simulink model "gm_soc_dvbs2_fpga"  (R2025b)
settings: Solver=VariableStepAuto  StartTime=0.0  StopTime=10.0  RelTol=1e-3
InitFcn:
  | soc_dvbs2_init;
undefined symbols (not defined in the file or in its folder): Add, coefficientsLog, coefficientsSqrt1, coefficientsSqrt2, dataBits, Deinterleaver, designMultirateFIR, noisePow, Shift, Short, soc_dvbs2_designFIRFilter, soc_dvbs2_txPacketBits, syncWord, txDataOut, txFiltCoeff, XData
libraries: simulink x304, hdlsllib x265, dspsigops x15, dsphdlfiltering2 x8, hdlmdlgenlib x6, dsphdlsigops2 x5, commseqgen3 x5, dsphdlmathfun2 x3, hwlogicconnlib x2, whdledac x2, commhdlcrc x2, whdlutilities x1
(part 35 of 36)

== system gm_soc_dvbs2_fpga/DVBS2/DVBS2 TxRx/DVB-S2 HDL Receiver/Synchronizer and PL Header Decoder/Time Frequency and Coarse Phase Synchronizer/Fine Frequency Synchronizer/Modified L and R Algorithm/L and R Algorithm 18 point/Compute R(m) for 7 to 12/Compute R(m)_1 ==
  z : Inport  OutDataTypeStr=fixdt(1, 16, 11)  PortDimensions=1  SampleTime=2.5e-07
      settings: SignalType=complex
  zvalid : Inport  Port=2  OutDataTypeStr=boolean  PortDimensions=1  SampleTime=2.5e-07
  Add3 : Sum  OutDataTypeStr=fixdt(1, 33, 22)  AccumDataTypeStr=fixdt(1, 34, 22)  SampleTime=2.5e-07
  Compare To Constant : simulink/Logic and Bit Operations/Compare To Constant  relop=>=  const="fi(0,0,6,0,\"hex\",\"07\")"  OutDataTypeStr=boolean
  Compare To Constant2 : simulink/Logic and Bit Operations/Compare To Constant  relop===  const="fi(0,0,6,0,\"hex\",\"23\")"  OutDataTypeStr=boolean
  Complex Multiplier : Subsystem
  Delay : Delay  DelayLength=double(7)  InitialCondition=0  SampleTime=2.5e-07
  Delay{1..2,7..9,11..12,14..15} (9 alike) : Delay  DelayLength=double(1)  InitialCondition=0  SampleTime=2.5e-07
  Delay{3..6,10,13,16..26} (17 alike) : Delay  DelayLength=double(2)  InitialCondition=0  SampleTime=2.5e-07
  Delay{27..30} (4 alike) : Delay  DelayLength=double(8)  InitialCondition=0  SampleTime=2.5e-07
  Gain : Gain  Gain="fi(0,0,16,20,\"hex\",\"8d3e\")"  ParamDataTypeStr=fixdt(0, 16, 20)  OutDataTypeStr=fixdt(1, 33, 22)  SampleTime=2.5e-07
  HDL Counter : hdlsllib/Sources/HDL Counter  CountType=Count limited  CountInit=0  CountStep=1  CountMax=N-1  CountFromType=Initial value  CountFrom=0  CountResetPort=off  CountLoadPort=off  CountEnbPort=on  CountDirPort=off  CountHitOutputPort=off  CountDataType=Unsigned  CountWordLen=nextpow2(N-1)  CountFracLen=0  CountSampTime=1
  Logical Operator : Logic  AllPortsSameDT=off  OutDataTypeStr=boolean  SampleTime=2.5e-07
  Logical Operator1 : Logic  AllPortsSameDT=off  OutDataTypeStr=boolean  SampleTime=2.5e-07
  Math Function : Math  Operator=conj  OutDataTypeStr=fixdt(1, 16, 11)
  Unit Delay Enabled Resettable Synchronous : hdlsllib/Discrete/Unit Delay Enabled Resettable Synchronous  InitialCondition=double(0)  SampleTime=-1
  Unit Delay Enabled Synchronous : hdlsllib/Discrete/Unit Delay Enabled Synchronous  InitialCondition=double(0)  SampleTime=-1
  Out1 : Outport  SampleTime=2.5e-07
  wires:
  Delay23/1 -> Delay24/1
  zvalid/1 -> Delay14/1
  Delay12/1 -> Delay6/1
  Logical Operator/1 -> Delay25/1
  Delay14/1 -> Delay15/1, Delay9/1, HDL Counter/1
  Delay9/1 -> Delay10/1
  Unit Delay Enabled Synchronous/1 -> Out1/1
  HDL Counter/1 -> Delay12/1, Delay11/1
  Math Function/1 -> Delay8/1
  Delay11/1 -> Delay5/1
  Delay15/1 -> Delay16/1
  Add3/1 -> Unit Delay Enabled Resettable Synchronous/1
  z/1 -> Delay2/1
  Delay16/1 -> Delay30/1
  Delay2/1 -> Delay7/1, Delay/1
  Logical Operator1/1 -> Delay23/1
  Delay10/1 -> Delay27/1
  Delay5/1 -> Delay28/1
  Delay6/1 -> Delay29/1
  Delay/1 -> Math Function/1
  Delay28/1 -> Compare To Constant/1
  Delay29/1 -> Compare To Constant2/1
  Delay30/1 -> Delay20/1
  Complex Multiplier/1(Out1) -> Delay13/1
  Delay7/1 -> Delay3/1
  Delay27/1 -> Delay17/1
  Compare To Constant2/1 -> Delay19/1
  Compare To Constant/1 -> Delay18/1
  Delay20/1 -> Logical Operator/2
  Delay8/1 -> Delay4/1
  Delay17/1 -> Logical Operator1/1
  Delay18/1 -> Logical Operator1/2
  Unit Delay Enabled Resettable Synchronous/1 -> Unit Delay Enabled Synchronous/1, Add3/1
  Delay19/1 -> Logical Operator/1
  Delay3/1 -> Complex Multiplier/1(In1)
  Delay4/1 -> Complex Multiplier/2(In2)
  Delay25/1 -> Delay26/1
  Delay13/1 -> Delay21/1
  Delay26/1 -> Delay1/1
  Delay21/1 -> Gain/1
  Delay24/1 -> Unit Delay Enabled Resettable Synchronous/2
  Delay1/1 -> Unit Delay Enabled Resettable Synchronous/3, Unit Delay Enabled Synchronous/2
  Gain/1 -> Delay22/1
  Delay22/1 -> Add3/2

== system gm_soc_dvbs2_fpga/DVBS2/DVBS2 TxRx/DVB-S2 HDL Receiver/Synchronizer and PL Header Decoder/Time Frequency and Coarse Phase Synchronizer/Fine Frequency Synchronizer/Modified L and R Algorithm/L and R Algorithm 18 point/Compute R(m) for 7 to 12/Compute R(m)_2 ==
  z : Inport  OutDataTypeStr=fixdt(1, 16, 11)  PortDimensions=1  SampleTime=2.5e-07
      settings: SignalType=complex
  zvalid : Inport  Port=2  OutDataTypeStr=boolean  PortDimensions=1  SampleTime=2.5e-07
  Add3 : Sum  OutDataTypeStr=fixdt(1, 33, 22)  AccumDataTypeStr=fixdt(1, 34, 22)  SampleTime=2.5e-07
  Compare To Constant : simulink/Logic and Bit Operations/Compare To Constant  relop=>=  const="fi(0,0,6,0,\"hex\",\"08\")"  OutDataTypeStr=boolean
  Compare To Constant2 : simulink/Logic and Bit Operations/Compare To Constant  relop===  const="fi(0,0,6,0,\"hex\",\"23\")"  OutDataTypeStr=boolean
  Complex Multiplier : Subsystem
  Delay{,27..30} (5 alike) : Delay  DelayLength=double(8)  InitialCondition=0  SampleTime=2.5e-07
  Delay{1..2,7..9,11..12,14..15} (9 alike) : Delay  DelayLength=double(1)  InitialCondition=0  SampleTime=2.5e-07
  Delay{3..6,10,13,16..26} (17 alike) : Delay  DelayLength=double(2)  InitialCondition=0  SampleTime=2.5e-07
  Gain : Gain  Gain="fi(0,0,16,20,\"hex\",\"9249\")"  ParamDataTypeStr=fixdt(0, 16, 20)  OutDataTypeStr=fixdt(1, 33, 22)  SampleTime=2.5e-07
  HDL Counter : hdlsllib/Sources/HDL Counter  CountType=Count limited  CountInit=0  CountStep=1  CountMax=N-1  CountFromType=Initial value  CountFrom=0  CountResetPort=off  CountLoadPort=off  CountEnbPort=on  CountDirPort=off  CountHitOutputPort=off  CountDataType=Unsigned  CountWordLen=nextpow2(N-1)  CountFracLen=0  CountSampTime=1
  Logical Operator : Logic  AllPortsSameDT=off  OutDataTypeStr=boolean  SampleTime=2.5e-07
  Logical Operator1 : Logic  AllPortsSameDT=off  OutDataTypeStr=boolean  SampleTime=2.5e-07
  Math Function : Math  Operator=conj  OutDataTypeStr=fixdt(1, 16, 11)
  Unit Delay Enabled Resettable Synchronous : hdlsllib/Discrete/Unit Delay Enabled Resettable Synchronous  InitialCondition=double(0)  SampleTime=-1
  Unit Delay Enabled Synchronous : hdlsllib/Discrete/Unit Delay Enabled Synchronous  InitialCondition=double(0)  SampleTime=-1
  Out1 : Outport  SampleTime=2.5e-07
  wires:
  Complex Multiplier/1(Out1) -> Delay13/1
  Delay12/1 -> Delay6/1
  Delay21/1 -> Gain/1
  Delay14/1 -> Delay9/1, Delay15/1, HDL Counter/1
  Logical Operator/1 -> Delay25/1
  Delay18/1 -> Logical Operator1/2
  zvalid/1 -> Delay14/1
  Delay9/1 -> Delay10/1
  HDL Counter/1 -> Delay11/1, Delay12/1
  z/1 -> Delay2/1
  Delay11/1 -> Delay5/1
  Delay22/1 -> Add3/2
  Math Function/1 -> Delay8/1
  Delay15/1 -> Delay16/1
  Delay16/1 -> Delay30/1
  Delay2/1 -> Delay7/1, Delay/1
  Delay10/1 -> Delay27/1
  Delay5/1 -> Delay28/1
  Delay6/1 -> Delay29/1
  Delay30/1 -> Delay20/1
  Delay23/1 -> Delay24/1
  Delay/1 -> Math Function/1
  Delay28/1 -> Compare To Constant/1
  Delay29/1 -> Compare To Constant2/1
  Delay7/1 -> Delay3/1
  Unit Delay Enabled Resettable Synchronous/1 -> Unit Delay Enabled Synchronous/1, Add3/1
  Delay27/1 -> Delay17/1
  Compare To Constant/1 -> Delay18/1
  Delay1/1 -> Unit Delay Enabled Synchronous/2, Unit Delay Enabled Resettable Synchronous/3
  Delay17/1 -> Logical Operator1/1
  Compare To Constant2/1 -> Delay19/1
  Delay3/1 -> Complex Multiplier/1(In1)
  Delay8/1 -> Delay4/1
  Add3/1 -> Unit Delay Enabled Resettable Synchronous/1
  Delay19/1 -> Logical Operator/1
  Delay20/1 -> Logical Operator/2
  Delay4/1 -> Complex Multiplier/2(In2)
  Logical Operator1/1 -> Delay23/1
  Delay25/1 -> Delay26/1
  Delay13/1 -> Delay21/1
  Delay26/1 -> Delay1/1
  Delay24/1 -> Unit Delay Enabled Resettable Synchronous/2
  Gain/1 -> Delay22/1
  Unit Delay Enabled Synchronous/1 -> Out1/1

== system gm_soc_dvbs2_fpga/DVBS2/DVBS2 TxRx/DVB-S2 HDL Receiver/Synchronizer and PL Header Decoder/Time Frequency and Coarse Phase Synchronizer/Fine Frequency Synchronizer/Modified L and R Algorithm/L and R Algorithm 18 point/Compute R(m) for 7 to 12/Compute R(m)_3 ==
  z : Inport  OutDataTypeStr=fixdt(1, 16, 11)  PortDimensions=1  SampleTime=2.5e-07
      settings: SignalType=complex
  zvalid : Inport  Port=2  OutDataTypeStr=boolean  PortDimensions=1  SampleTime=2.5e-07
  Add3 : Sum  OutDataTypeStr=fixdt(1, 33, 22)  AccumDataTypeStr=fixdt(1, 34, 22)  SampleTime=2.5e-07
  Compare To Constant : simulink/Logic and Bit Operations/Compare To Constant  relop=>=  const="fi(0,0,6,0,\"hex\",\"09\")"  OutDataTypeStr=boolean
  Compare To Constant2 : simulink/Logic and Bit Operations/Compare To Constant  relop===  const="fi(0,0,6,0,\"hex\",\"23\")"  OutDataTypeStr=boolean
  Complex Multiplier : Subsystem
  Delay : Delay  DelayLength=double(9)  InitialCondition=0  SampleTime=2.5e-07
  Delay{1..2,7..9,11..12,14..15} (9 alike) : Delay  DelayLength=double(1)  InitialCondition=0  SampleTime=2.5e-07
  Delay{3..6,10,13,16..26} (17 alike) : Delay  DelayLength=double(2)  InitialCondition=0  SampleTime=2.5e-07
  Delay{27..30} (4 alike) : Delay  DelayLength=double(8)  InitialCondition=0  SampleTime=2.5e-07
  Gain : Gain  Gain="fi(0,0,16,20,\"hex\",\"97b4\")"  ParamDataTypeStr=fixdt(0, 16, 20)  OutDataTypeStr=fixdt(1, 33, 22)  SampleTime=2.5e-07
  HDL Counter : hdlsllib/Sources/HDL Counter  CountType=Count limited  CountInit=0  CountStep=1  CountMax=N-1  CountFromType=Initial value  CountFrom=0  CountResetPort=off  CountLoadPort=off  CountEnbPort=on  CountDirPort=off  CountHitOutputPort=off  CountDataType=Unsigned  CountWordLen=nextpow2(N-1)  CountFracLen=0  CountSampTime=1
  Logical Operator : Logic  AllPortsSameDT=off  OutDataTypeStr=boolean  SampleTime=2.5e-07
  Logical Operator1 : Logic  AllPortsSameDT=off  OutDataTypeStr=boolean  SampleTime=2.5e-07
  Math Function : Math  Operator=conj  OutDataTypeStr=fixdt(1, 16, 11)
  Unit Delay Enabled Resettable Synchronous : hdlsllib/Discrete/Unit Delay Enabled Resettable Synchronous  InitialCondition=double(0)  SampleTime=-1
  Unit Delay Enabled Synchronous : hdlsllib/Discrete/Unit Delay Enabled Synchronous  InitialCondition=double(0)  SampleTime=-1
  Out1 : Outport  SampleTime=2.5e-07
  wires:
  zvalid/1 -> Delay14/1
  Logical Operator/1 -> Delay25/1
  Delay10/1 -> Delay27/1
  Logical Operator1/1 -> Delay23/1
  Delay14/1 -> Delay15/1, Delay9/1, HDL Counter/1
  Delay9/1 -> Delay10/1
  HDL Counter/1 -> Delay12/1, Delay11/1
  Add3/1 -> Unit Delay Enabled Resettable Synchronous/1
  Delay11/1 -> Delay5/1
  Delay15/1 -> Delay16/1
  z/1 -> Delay2/1
  Delay12/1 -> Delay6/1
  Delay16/1 -> Delay30/1
  Delay2/1 -> Delay7/1, Delay/1
  Delay27/1 -> Delay17/1
  Delay5/1 -> Delay28/1
  Delay6/1 -> Delay29/1
  Delay30/1 -> Delay20/1
  Delay/1 -> Math Function/1
  Delay28/1 -> Compare To Constant/1
  Delay29/1 -> Compare To Constant2/1
  Delay7/1 -> Delay3/1
  Math Function/1 -> Delay8/1
  Compare To Constant2/1 -> Delay19/1
  Compare To Constant/1 -> Delay18/1
  Delay20/1 -> Logical Operator/2
  Delay3/1 -> Complex Multiplier/1(In1)
  Delay8/1 -> Delay4/1
  Delay1/1 -> Unit Delay Enabled Synchronous/2, Unit Delay Enabled Resettable Synchronous/3
  Delay17/1 -> Logical Operator1/1
  Delay18/1 -> Logical Operator1/2
  Delay19/1 -> Logical Operator/1
  Delay4/1 -> Complex Multiplier/2(In2)
  Complex Multiplier/1(Out1) -> Delay13/1
  Delay25/1 -> Delay26/1
  Delay13/1 -> Delay21/1
  Delay23/1 -> Delay24/1
  Delay26/1 -> Delay1/1
  Delay21/1 -> Gain/1
  Delay24/1 -> Unit Delay Enabled Resettable Synchronous/2
  Gain/1 -> Delay22/1
  Delay22/1 -> Add3/2
  Unit Delay Enabled Resettable Synchronous/1 -> Unit Delay Enabled Synchronous/1, Add3/1
  Unit Delay Enabled Synchronous/1 -> Out1/1

== system gm_soc_dvbs2_fpga/DVBS2/DVBS2 TxRx/DVB-S2 HDL Receiver/Synchronizer and PL Header Decoder/Time Frequency and Coarse Phase Synchronizer/Fine Frequency Synchronizer/Modified L and R Algorithm/L and R Algorithm 18 point/Compute R(m) for 7 to 12/Compute R(m)_4 ==
  z : Inport  OutDataTypeStr=fixdt(1, 16, 11)  PortDimensions=1  SampleTime=2.5e-07
      settings: SignalType=complex
  zvalid : Inport  Port=2  OutDataTypeStr=boolean  PortDimensions=1  SampleTime=2.5e-07
  Add3 : Sum  OutDataTypeStr=fixdt(1, 33, 22)  AccumDataTypeStr=fixdt(1, 34, 22)  SampleTime=2.5e-07
  Compare To Constant : simulink/Logic and Bit Operations/Compare To Constant  relop=>=  const="fi(0,0,6,0,\"hex\",\"0a\")"  OutDataTypeStr=boolean
  Compare To Constant2 : simulink/Logic and Bit Operations/Compare To Constant  relop===  const="fi(0,0,6,0,\"hex\",\"23\")"  OutDataTypeStr=boolean
  Complex Multiplier : Subsystem
  Delay : Delay  DelayLength=double(10)  InitialCondition=0  SampleTime=2.5e-07
  Delay{1..2,7..9,11..12,14..15} (9 alike) : Delay  DelayLength=double(1)  InitialCondition=0  SampleTime=2.5e-07
  Delay{3..6,10,13,16..26} (17 alike) : Delay  DelayLength=double(2)  InitialCondition=0  SampleTime=2.5e-07
  Delay{27..30} (4 alike) : Delay  DelayLength=double(8)  InitialCondition=0  SampleTime=2.5e-07
  Gain : Gain  Gain="fi(0,0,16,20,\"hex\",\"9d8a\")"  ParamDataTypeStr=fixdt(0, 16, 20)  OutDataTypeStr=fixdt(1, 33, 22)  SampleTime=2.5e-07
  HDL Counter : hdlsllib/Sources/HDL Counter  CountType=Count limited  CountInit=0  CountStep=1  CountMax=N-1  CountFromType=Initial value  CountFrom=0  CountResetPort=off  CountLoadPort=off  CountEnbPort=on  CountDirPort=off  CountHitOutputPort=off  CountDataType=Unsigned  CountWordLen=nextpow2(N-1)  CountFracLen=0  CountSampTime=1
  Logical Operator : Logic  AllPortsSameDT=off  OutDataTypeStr=boolean  SampleTime=2.5e-07
  Logical Operator1 : Logic  AllPortsSameDT=off  OutDataTypeStr=boolean  SampleTime=2.5e-07
  Math Function : Math  Operator=conj  OutDataTypeStr=fixdt(1, 16, 11)
  Unit Delay Enabled Resettable Synchronous : hdlsllib/Discrete/Unit Delay Enabled Resettable Synchronous  InitialCondition=double(0)  SampleTime=-1
  Unit Delay Enabled Synchronous : hdlsllib/Discrete/Unit Delay Enabled Synchronous  InitialCondition=double(0)  SampleTime=-1
  Out1 : Outport  SampleTime=2.5e-07
  wires:
  Delay10/1 -> Delay27/1
  Delay21/1 -> Gain/1
  Delay14/1 -> Delay9/1, Delay15/1, HDL Counter/1
  Delay12/1 -> Delay6/1
  zvalid/1 -> Delay14/1
  Delay9/1 -> Delay10/1
  HDL Counter/1 -> Delay12/1, Delay11/1
  Delay11/1 -> Delay5/1
  Delay20/1 -> Logical Operator/2
  z/1 -> Delay2/1
  Delay22/1 -> Add3/2
  Math Function/1 -> Delay8/1
  Delay15/1 -> Delay16/1
  Delay16/1 -> Delay30/1
  Delay2/1 -> Delay7/1, Delay/1
  Delay27/1 -> Delay17/1
  Delay5/1 -> Delay28/1
  Delay6/1 -> Delay29/1
  Delay30/1 -> Delay20/1
  Delay7/1 -> Delay3/1
  Delay/1 -> Math Function/1
  Delay28/1 -> Compare To Constant/1
  Delay29/1 -> Compare To Constant2/1
  Delay3/1 -> Complex Multiplier/1(In1)
  Compare To Constant/1 -> Delay18/1
  Delay17/1 -> Logical Operator1/1
  Compare To Constant2/1 -> Delay19/1
  Delay8/1 -> Delay4/1
  Complex Multiplier/1(Out1) -> Delay13/1
  Logical Operator/1 -> Delay25/1
  Delay18/1 -> Logical Operator1/2
  Add3/1 -> Unit Delay Enabled Resettable Synchronous/1
  Delay19/1 -> Logical Operator/1
  Delay4/1 -> Complex Multiplier/2(In2)
  Logical Operator1/1 -> Delay23/1
  Delay25/1 -> Delay26/1
  Delay13/1 -> Delay21/1
  Delay23/1 -> Delay24/1
  Delay26/1 -> Delay1/1
  Delay24/1 -> Unit Delay Enabled Resettable Synchronous/2
  Delay1/1 -> Unit Delay Enabled Synchronous/2, Unit Delay Enabled Resettable Synchronous/3
  Gain/1 -> Delay22/1
  Unit Delay Enabled Resettable Synchronous/1 -> Unit Delay Enabled Synchronous/1, Add3/1
  Unit Delay Enabled Synchronous/1 -> Out1/1

== system gm_soc_dvbs2_fpga/DVBS2/DVBS2 TxRx/DVB-S2 HDL Receiver/Synchronizer and PL Header Decoder/Time Frequency and Coarse Phase Synchronizer/Fine Frequency Synchronizer/Modified L and R Algorithm/L and R Algorithm 18 point/Compute R(m) for 7 to 12/Compute R(m)_5 ==
  z : Inport  OutDataTypeStr=fixdt(1, 16, 11)  PortDimensions=1  SampleTime=2.5e-07
      settings: SignalType=complex
  zvalid : Inport  Port=2  OutDataTypeStr=boolean  PortDimensions=1  SampleTime=2.5e-07
  Add3 : Sum  OutDataTypeStr=fixdt(1, 33, 22)  AccumDataTypeStr=fixdt(1, 34, 22)  SampleTime=2.5e-07
  Compare To Constant : simulink/Logic and Bit Operations/Compare To Constant  relop=>=  const="fi(0,0,6,0,\"hex\",\"0b\")"  OutDataTypeStr=boolean
  Compare To Constant2 : simulink/Logic and Bit Operations/Compare To Constant  relop===  const="fi(0,0,6,0,\"hex\",\"23\")"  OutDataTypeStr=boolean
  Complex Multiplier : Subsystem
  Delay : Delay  DelayLength=double(11)  InitialCondition=0  SampleTime=2.5e-07
  Delay{1..2,7..9,11..12,14..15} (9 alike) : Delay  DelayLength=double(1)  InitialCondition=0  SampleTime=2.5e-07
  Delay{3..6,10,13,16..26} (17 alike) : Delay  DelayLength=double(2)  InitialCondition=0  SampleTime=2.5e-07
  Delay{27..30} (4 alike) : Delay  DelayLength=double(8)  InitialCondition=0  SampleTime=2.5e-07
  Gain : Gain  Gain="fi(0,0,16,20,\"hex\",\"a3d7\")"  ParamDataTypeStr=fixdt(0, 16, 20)  OutDataTypeStr=fixdt(1, 33, 22)  SampleTime=2.5e-07
  HDL Counter : hdlsllib/Sources/HDL Counter  CountType=Count limited  CountInit=0  CountStep=1  CountMax=N-1  CountFromType=Initial value  CountFrom=0  CountResetPort=off  CountLoadPort=off  CountEnbPort=on  CountDirPort=off  CountHitOutputPort=off  CountDataType=Unsigned  CountWordLen=nextpow2(N-1)  CountFracLen=0  CountSampTime=1
  Logical Operator : Logic  AllPortsSameDT=off  OutDataTypeStr=boolean  SampleTime=2.5e-07
  Logical Operator1 : Logic  AllPortsSameDT=off  OutDataTypeStr=boolean  SampleTime=2.5e-07
  Math Function : Math  Operator=conj  OutDataTypeStr=fixdt(1, 16, 11)
  Unit Delay Enabled Resettable Synchronous : hdlsllib/Discrete/Unit Delay Enabled Resettable Synchronous  InitialCondition=double(0)  SampleTime=-1
  Unit Delay Enabled Synchronous : hdlsllib/Discrete/Unit Delay Enabled Synchronous  InitialCondition=double(0)  SampleTime=-1
  Out1 : Outport  SampleTime=2.5e-07
  wires:
  zvalid/1 -> Delay14/1
  Logical Operator1/1 -> Delay23/1
  Delay10/1 -> Delay27/1
  Logical Operator/1 -> Delay25/1
  Delay14/1 -> Delay9/1, Delay15/1, HDL Counter/1
  Delay9/1 -> Delay10/1
  Unit Delay Enabled Synchronous/1 -> Out1/1
  HDL Counter/1 -> Delay12/1, Delay11/1
  Math Function/1 -> Delay8/1
  Delay11/1 -> Delay5/1
  Delay15/1 -> Delay16/1
  z/1 -> Delay2/1
  Delay12/1 -> Delay6/1
  Delay16/1 -> Delay30/1
  Delay2/1 -> Delay7/1, Delay/1
  Delay27/1 -> Delay17/1
  Delay5/1 -> Delay28/1
  Delay6/1 -> Delay29/1
  Delay/1 -> Math Function/1
  Delay28/1 -> Compare To Constant/1
  Delay29/1 -> Compare To Constant2/1
  Delay30/1 -> Delay20/1
  Delay7/1 -> Delay3/1
  Delay20/1 -> Logical Operator/2
  Compare To Constant2/1 -> Delay19/1
  Compare To Constant/1 -> Delay18/1
  Delay3/1 -> Complex Multiplier/1(In1)
  Delay8/1 -> Delay4/1
  Delay1/1 -> Unit Delay Enabled Synchronous/2, Unit Delay Enabled Resettable Synchronous/3
  Delay17/1 -> Logical Operator1/1
  Delay18/1 -> Logical Operator1/2
  Delay19/1 -> Logical Operator/1
  Delay4/1 -> Complex Multiplier/2(In2)
  Complex Multiplier/1(Out1) -> Delay13/1
  Delay25/1 -> Delay26/1
  Delay13/1 -> Delay21/1
  Delay24/1 -> Unit Delay Enabled Resettable Synchronous/2
  Delay23/1 -> Delay24/1
  Delay26/1 -> Delay1/1
  Delay21/1 -> Gain/1
  Gain/1 -> Delay22/1
  Unit Delay Enabled Resettable Synchronous/1 -> Unit Delay Enabled Synchronous/1, Add3/1
  Delay22/1 -> Add3/2
  Add3/1 -> Unit Delay Enabled Resettable Synchronous/1

== system gm_soc_dvbs2_fpga/DVBS2/DVBS2 TxRx/DVB-S2 HDL Receiver/Synchronizer and PL Header Decoder/Time Frequency and Coarse Phase Synchronizer/Fine Frequency Synchronizer/Modified L and R Algorithm/L and R Algorithm 18 point/Compute R(m) for 7 to 12/Compute R(m)_6 ==
  z : Inport  OutDataTypeStr=fixdt(1, 16, 11)  PortDimensions=1  SampleTime=2.5e-07
      settings: SignalType=complex
  zvalid : Inport  Port=2  OutDataTypeStr=boolean  PortDimensions=1  SampleTime=2.5e-07
  Add3 : Sum  OutDataTypeStr=fixdt(1, 33, 22)  AccumDataTypeStr=fixdt(1, 34, 22)  SampleTime=2.5e-07
  Compare To Constant : simulink/Logic and Bit Operations/Compare To Constant  relop=>=  const="fi(0,0,6,0,\"hex\",\"0c\")"  OutDataTypeStr=boolean
  Compare To Constant2 : simulink/Logic and Bit Operations/Compare To Constant  relop===  const="fi(0,0,6,0,\"hex\",\"23\")"  OutDataTypeStr=boolean
  Complex Multiplier : Subsystem
  Delay : Delay  DelayLength=double(12)  InitialCondition=0  SampleTime=2.5e-07
  Delay{1..2,7..9,11..12,14..15} (9 alike) : Delay  DelayLength=double(1)  InitialCondition=0  SampleTime=2.5e-07
  Delay{3..6,10,13,16..26} (17 alike) : Delay  DelayLength=double(2)  InitialCondition=0  SampleTime=2.5e-07
  Delay{27..30} (4 alike) : Delay  DelayLength=double(8)  InitialCondition=0  SampleTime=2.5e-07
  Gain : Gain  Gain="fi(0,0,16,20,\"hex\",\"aaab\")"  ParamDataTypeStr=fixdt(0, 16, 20)  OutDataTypeStr=fixdt(1, 33, 22)  SampleTime=2.5e-07
  HDL Counter : hdlsllib/Sources/HDL Counter  CountType=Count limited  CountInit=0  CountStep=1  CountMax=N-1  CountFromType=Initial value  CountFrom=0  CountResetPort=off  CountLoadPort=off  CountEnbPort=on  CountDirPort=off  CountHitOutputPort=off  CountDataType=Unsigned  CountWordLen=nextpow2(N-1)  CountFracLen=0  CountSampTime=1
  Logical Operator : Logic  AllPortsSameDT=off  OutDataTypeStr=boolean  SampleTime=2.5e-07
  Logical Operator1 : Logic  AllPortsSameDT=off  OutDataTypeStr=boolean  SampleTime=2.5e-07
  Math Function : Math  Operator=conj  OutDataTypeStr=fixdt(1, 16, 11)
  Unit Delay Enabled Resettable Synchronous : hdlsllib/Discrete/Unit Delay Enabled Resettable Synchronous  InitialCondition=double(0)  SampleTime=-1
  Unit Delay Enabled Synchronous : hdlsllib/Discrete/Unit Delay Enabled Synchronous  InitialCondition=double(0)  SampleTime=-1
  Out1 : Outport  SampleTime=2.5e-07
  wires:
  Delay21/1 -> Gain/1
  Delay14/1 -> Delay9/1, Delay15/1, HDL Counter/1
  Delay23/1 -> Delay24/1
  zvalid/1 -> Delay14/1
  Delay9/1 -> Delay10/1
  HDL Counter/1 -> Delay12/1, Delay11/1
  Delay17/1 -> Logical Operator1/1
  z/1 -> Delay2/1
  Add3/1 -> Unit Delay Enabled Resettable Synchronous/1
  Delay22/1 -> Add3/2
  Delay15/1 -> Delay16/1
  Delay11/1 -> Delay5/1
  Delay12/1 -> Delay6/1
  Delay16/1 -> Delay30/1
  Delay2/1 -> Delay7/1, Delay/1
  Delay10/1 -> Delay27/1
  Delay5/1 -> Delay28/1
  Delay6/1 -> Delay29/1
  Delay7/1 -> Delay3/1
  Delay/1 -> Math Function/1
  Delay27/1 -> Delay17/1
  Delay28/1 -> Compare To Constant/1
  Delay29/1 -> Compare To Constant2/1
  Delay30/1 -> Delay20/1
  Delay19/1 -> Logical Operator/1
  Math Function/1 -> Delay8/1
  Compare To Constant2/1 -> Delay19/1
  Compare To Constant/1 -> Delay18/1
  Delay3/1 -> Complex Multiplier/1(In1)
  Delay8/1 -> Delay4/1
  Logical Operator1/1 -> Delay23/1
  Delay18/1 -> Logical Operator1/2
  Delay20/1 -> Logical Operator/2
  Delay4/1 -> Complex Multiplier/2(In2)
  Logical Operator/1 -> Delay25/1
  Complex Multiplier/1(Out1) -> Delay13/1
  Delay25/1 -> Delay26/1
  Delay13/1 -> Delay21/1
  Delay26/1 -> Delay1/1
  Delay24/1 -> Unit Delay Enabled Resettable Synchronous/2
  Delay1/1 -> Unit Delay Enabled Synchronous/2, Unit Delay Enabled Resettable Synchronous/3
  Gain/1 -> Delay22/1
  Unit Delay Enabled Resettable Synchronous/1 -> Unit Delay Enabled Synchronous/1, Add3/1
  Unit Delay Enabled Synchronous/1 -> Out1/1

== system gm_soc_dvbs2_fpga/DVBS2/DVBS2 TxRx/DVB-S2 HDL Receiver/Synchronizer and PL Header Decoder/Time Frequency and Coarse Phase Synchronizer/Time and Coarse Frequency Synchronizer/PL Data Descrambler and Pilot Valid Indicator/PL Data Descrambler/PL Scrambler Gold Sequence Generator/Subsystem ==
  reset : Inport  OutDataTypeStr=boolean  PortDimensions=1  SampleTime=2.5e-07
  Enable : EnablePort  OutDataTypeStr=boolean
  X PN Generator M_n : commseqgen3/PN Sequence Generator  poly='z^18+z^7+1'  ini_sta=[zeros(1,17) 1]  outBitMaskSource=Dialog parameter  shift=n  outVarSiz=off  maxOutSizeMode=Dialog parameter  maxOutSize=[10 1]  Ts=-1  sampPerFrame=1  reset=on  bitPackedOutputs=off  outDataType=boolean  numPackedBits=8  bitPackDataSigned=off  bitPackedOutDType=double
  X PN Generator M_nplus131072 : commseqgen3/PN Sequence Generator  poly='z^18+z^7+1'  ini_sta=[zeros(1,17) 1]  outBitMaskSource=Dialog parameter  shift=n+131072  outVarSiz=off  maxOutSizeMode=Dialog parameter  maxOutSize=[10 1]  Ts=-1  sampPerFrame=1  reset=on  bitPackedOutputs=off  outDataType=boolean  numPackedBits=8  bitPackDataSigned=off  bitPackedOutDType=double
  Y PN Generator M_0 : commseqgen3/PN Sequence Generator  poly='z^18 + z^10 + z^7 + z^5 + 1'  ini_sta=ones(1,18)  outBitMaskSource=Dialog parameter  shift=0  outVarSiz=off  maxOutSizeMode=Dialog parameter  maxOutSize=[10 1]  Ts=-1  sampPerFrame=1  reset=on  bitPackedOutputs=off  outDataType=boolean  numPackedBits=8  bitPackDataSigned=off  bitPackedOutDType=double
  Y PN Generator M_131072 : commseqgen3/PN Sequence Generator  poly='z^18 + z^10 + z^7 + z^5 + 1'  ini_sta=ones(1,18)  outBitMaskSource=Dialog parameter  shift=131072  outVarSiz=off  maxOutSizeMode=Dialog parameter  maxOutSize=[10 1]  Ts=-1  sampPerFrame=1  reset=on  bitPackedOutputs=off  outDataType=boolean  numPackedBits=8  bitPackDataSigned=off  bitPackedOutDType=double
  xMnp131072 : Outport  SampleTime=2.5e-07  InitialOutput=0
  yM131072 : Outport  Port=2  SampleTime=2.5e-07  InitialOutput=0
  xMn : Outport  Port=3  SampleTime=2.5e-07  InitialOutput=0
  yM0 : Outport  Port=4  SampleTime=2.5e-07  InitialOutput=0
  wires:
  Y PN Generator M_0/1 -> yM0/1
  X PN Generator M_n/1 -> xMn/1
  reset/1 -> X PN Generator M_n/1, X PN Generator M_nplus131072/1, Y PN Generator M_0/1, Y PN Generator M_131072/1
  Y PN Generator M_131072/1 -> yM131072/1
  X PN Generator M_nplus131072/1 -> xMnp131072/1

== system gm_soc_dvbs2_fpga/DVBS2/DVBS2 TxRx/DVB-S2 HDL Receiver/Synchronizer and PL Header Decoder/Time Frequency and Coarse Phase Synchronizer/Time and Coarse Frequency Synchronizer/Symbol Synchronizer/Rate Handle/FIFO/MATLAB Function ==
  wr : Inport  OutDataTypeStr=boolean  PortDimensions=1  SampleTime=6.25e-08
  rd : Inport  Port=2  OutDataTypeStr=boolean  PortDimensions=1  SampleTime=6.25e-08
  MATLAB Function : MATLAB Function  TreatAsAtomicUnit=on
  full : Outport  SampleTime=6.25e-08  VectorParamsAs1DForOutWhenUnconnected=off
  empty : Outport  Port=2  SampleTime=6.25e-08
  wires:
  MATLAB Function/2(empty) -> empty/1
  MATLAB Function/1(full) -> full/1
  wr/1 -> MATLAB Function/1(wr)
  rd/1 -> MATLAB Function/2(rd)

== system gm_soc_dvbs2_fpga/DVBS2/DVBS2 TxRx/DVB-S2 HDL Receiver/Synchronizer and PL Header Decoder/Time Frequency and Coarse Phase Synchronizer/Fine Frequency Synchronizer/Modified L and R Algorithm/L and R Algorithm 18 point/Compute R(m) for 1 to 6/Compute R(m)_1/Complex Multiplier ==
  In1 : Inport  OutDataTypeStr=fixdt(1, 16, 11)  PortDimensions=1  SampleTime=2.5e-07
      settings: SignalType=complex
  In2 : Inport  Port=2  OutDataTypeStr=fixdt(1, 16, 11)  PortDimensions=1  SampleTime=2.5e-07
      settings: SignalType=complex
  AddADn : Sum  Inputs=++|  OutDataTypeStr=fixdt(1, 33, 22)
  AddAUp : Sum  Inputs=|+-  OutDataTypeStr=fixdt(1, 33, 22)
  AddBCtr : Sum  Inputs=+|+  OutDataTypeStr=fixdt(1, 17, 11)
  AddBDn : Sum  Inputs=|+-  OutDataTypeStr=fixdt(1, 17, 11)
  AddBUp : Sum  Inputs=++|  OutDataTypeStr=fixdt(1, 17, 11)
  Complex to Real-Imag : ComplexToRealImag
  Complex to Real-Imag1 : ComplexToRealImag
  Delay{1..5,8..20} (18 alike) : Delay  DelayLength=1
  Delay{6..7,21..27} (9 alike) : Delay
  Product : Product  OutDataTypeStr=fixdt(1, 33, 22)
  Product1 : Product  OutDataTypeStr=fixdt(1, 33, 22)
  Product2 : Product  OutDataTypeStr=fixdt(1, 33, 22)
  Real-Imag to Complex : RealImagToComplex
  Out1 : Outport  SampleTime=2.5e-07  VectorParamsAs1DForOutWhenUnconnected=off
  wires:
  Delay9/1 -> AddBUp/1
  Product2/1 -> Delay27/1
  Delay7/1 -> Product/2
  AddBDn/1 -> Delay5/1
  [IM2] -> Delay15/1
  [RE2] -> Delay14/1
  Delay5/1 -> Delay24/1
  [IM2] -> Delay10/1
  AddAUp/1 -> Delay19/1
  Product/1 -> Delay25/1
  [RE2] -> Delay9/1
  In1/1 -> Complex to Real-Imag/1
  In2/1 -> Complex to Real-Imag1/1
  Delay25/1 -> Delay16/1
  Delay10/1 -> AddBUp/2
  Complex to Real-Imag/1 -> Delay11/1
  Complex to Real-Imag/2 -> Delay13/1
  Complex to Real-Imag1/1 -> [RE2]
  Complex to Real-Imag1/2 -> [IM2]
  Delay14/1 -> AddBDn/1
  Delay15/1 -> AddBDn/2
  AddBUp/1 -> Delay8/1
  Delay26/1 -> Delay17/1
  Delay11/1 -> AddBCtr/1, Delay1/1
  Product1/1 -> Delay26/1
  AddBCtr/1 -> Delay2/1
  [IM2] -> Delay12/1
  Delay13/1 -> AddBCtr/2, Delay4/1
  Delay8/1 -> Delay6/1
  Delay24/1 -> Product2/2
  Delay1/1 -> Delay7/1
  Delay27/1 -> Delay18/1
  Delay12/1 -> Delay3/1
  Delay4/1 -> Delay23/1
  Delay6/1 -> Product/1
  Delay2/1 -> Delay21/1
  AddADn/1 -> Delay20/1
  Delay3/1 -> Delay22/1
  Delay23/1 -> Product2/1
  Delay21/1 -> Product1/1
  Delay22/1 -> Product1/2
  Delay16/1 -> AddAUp/1
  Delay17/1 -> AddAUp/2, AddADn/1
  Delay18/1 -> AddADn/2
  Delay19/1 -> Real-Imag to Complex/1
  Delay20/1 -> Real-Imag to Complex/2
  Real-Imag to Complex/1 -> Out1/1

== system gm_soc_dvbs2_fpga/DVBS2/DVBS2 TxRx/DVB-S2 HDL Receiver/Synchronizer and PL Header Decoder/Time Frequency and Coarse Phase Synchronizer/Fine Frequency Synchronizer/Modified L and R Algorithm/L and R Algorithm 18 point/Compute R(m) for 1 to 6/Compute R(m)_2/Complex Multiplier ==
  In1 : Inport  OutDataTypeStr=fixdt(1, 16, 11)  PortDimensions=1  SampleTime=2.5e-07
      settings: SignalType=complex
  In2 : Inport  Port=2  OutDataTypeStr=fixdt(1, 16, 11)  PortDimensions=1  SampleTime=2.5e-07
      settings: SignalType=complex
  AddADn : Sum  Inputs=++|  OutDataTypeStr=fixdt(1, 33, 22)
  AddAUp : Sum  Inputs=|+-  OutDataTypeStr=fixdt(1, 33, 22)
  AddBCtr : Sum  Inputs=+|+  OutDataTypeStr=fixdt(1, 17, 11)
  AddBDn : Sum  Inputs=|+-  OutDataTypeStr=fixdt(1, 17, 11)
  AddBUp : Sum  Inputs=++|  OutDataTypeStr=fixdt(1, 17, 11)
  Complex to Real-Imag : ComplexToRealImag
  Complex to Real-Imag1 : ComplexToRealImag
  Delay{1..5,8..20} (18 alike) : Delay  DelayLength=1
  Delay{6..7,21..27} (9 alike) : Delay
  Product : Product  OutDataTypeStr=fixdt(1, 33, 22)
  Product1 : Product  OutDataTypeStr=fixdt(1, 33, 22)
  Product2 : Product  OutDataTypeStr=fixdt(1, 33, 22)
  Real-Imag to Complex : RealImagToComplex
  Out1 : Outport  SampleTime=2.5e-07  VectorParamsAs1DForOutWhenUnconnected=off
  wires:
  Delay9/1 -> AddBUp/1
  Delay7/1 -> Product/2
  [IM2] -> Delay15/1
  Delay26/1 -> Delay17/1
  [RE2] -> Delay14/1
  Delay5/1 -> Delay24/1
  [IM2] -> Delay10/1
  Delay24/1 -> Product2/2
  [RE2] -> Delay9/1
  Delay11/1 -> AddBCtr/1, Delay1/1
  In1/1 -> Complex to Real-Imag/1
  Delay10/1 -> AddBUp/2
  Delay12/1 -> Delay3/1
  In2/1 -> Complex to Real-Imag1/1
  Complex to Real-Imag/1 -> Delay11/1
  AddAUp/1 -> Delay19/1
  Product/1 -> Delay25/1
  Complex to Real-Imag/2 -> Delay13/1
  Complex to Real-Imag1/1 -> [RE2]
  Product1/1 -> Delay26/1
  AddBCtr/1 -> Delay2/1
  Complex to Real-Imag1/2 -> [IM2]
  Delay14/1 -> AddBDn/1
  Delay15/1 -> AddBDn/2
  AddADn/1 -> Delay20/1
  AddBUp/1 -> Delay8/1
  Delay20/1 -> Real-Imag to Complex/2
  [IM2] -> Delay12/1
  Delay13/1 -> AddBCtr/2, Delay4/1
  Real-Imag to Complex/1 -> Out1/1
  Product2/1 -> Delay27/1
  AddBDn/1 -> Delay5/1
  Delay8/1 -> Delay6/1
  Delay1/1 -> Delay7/1
  Delay4/1 -> Delay23/1
  Delay6/1 -> Product/1
  Delay2/1 -> Delay21/1
  Delay3/1 -> Delay22/1
  Delay23/1 -> Product2/1
  Delay21/1 -> Product1/1
  Delay22/1 -> Product1/2
  Delay25/1 -> Delay16/1
  Delay27/1 -> Delay18/1
  Delay16/1 -> AddAUp/1
  Delay17/1 -> AddADn/1, AddAUp/2
  Delay18/1 -> AddADn/2
  Delay19/1 -> Real-Imag to Complex/1

== system gm_soc_dvbs2_fpga/DVBS2/DVBS2 TxRx/DVB-S2 HDL Receiver/Synchronizer and PL Header Decoder/Time Frequency and Coarse Phase Synchronizer/Fine Frequency Synchronizer/Modified L and R Algorithm/L and R Algorithm 18 point/Compute R(m) for 1 to 6/Compute R(m)_3/Complex Multiplier ==
  In1 : Inport  OutDataTypeStr=fixdt(1, 16, 11)  PortDimensions=1  SampleTime=2.5e-07
      settings: SignalType=complex
  In2 : Inport  Port=2  OutDataTypeStr=fixdt(1, 16, 11)  PortDimensions=1  SampleTime=2.5e-07
      settings: SignalType=complex
  AddADn : Sum  Inputs=++|  OutDataTypeStr=fixdt(1, 33, 22)
  AddAUp : Sum  Inputs=|+-  OutDataTypeStr=fixdt(1, 33, 22)
  AddBCtr : Sum  Inputs=+|+  OutDataTypeStr=fixdt(1, 17, 11)
  AddBDn : Sum  Inputs=|+-  OutDataTypeStr=fixdt(1, 17, 11)
  AddBUp : Sum  Inputs=++|  OutDataTypeStr=fixdt(1, 17, 11)
  Complex to Real-Imag : ComplexToRealImag
  Complex to Real-Imag1 : ComplexToRealImag
  Delay{1..5,8..20} (18 alike) : Delay  DelayLength=1
  Delay{6..7,21..27} (9 alike) : Delay
  Product : Product  OutDataTypeStr=fixdt(1, 33, 22)
  Product1 : Product  OutDataTypeStr=fixdt(1, 33, 22)
  Product2 : Product  OutDataTypeStr=fixdt(1, 33, 22)
  Real-Imag to Complex : RealImagToComplex
  Out1 : Outport  SampleTime=2.5e-07  VectorParamsAs1DForOutWhenUnconnected=off
  wires:
  Delay9/1 -> AddBUp/1
  Product2/1 -> Delay27/1
  Delay7/1 -> Product/2
  AddBDn/1 -> Delay5/1
  [IM2] -> Delay15/1
  [RE2] -> Delay14/1
  [IM2] -> Delay10/1
  AddAUp/1 -> Delay19/1
  Product/1 -> Delay25/1
  Complex to Real-Imag/2 -> Delay13/1
  [RE2] -> Delay9/1
  In1/1 -> Complex to Real-Imag/1
  In2/1 -> Complex to Real-Imag1/1
  Delay18/1 -> AddADn/2
  Delay10/1 -> AddBUp/2
  Complex to Real-Imag/1 -> Delay11/1
  Complex to Real-Imag1/1 -> [RE2]
  Complex to Real-Imag1/2 -> [IM2]
  Delay14/1 -> AddBDn/1
  Delay15/1 -> AddBDn/2
  AddADn/1 -> Delay20/1
  AddBUp/1 -> Delay8/1
  Delay19/1 -> Real-Imag to Complex/1
  Delay11/1 -> AddBCtr/1, Delay1/1
  Product1/1 -> Delay26/1
  AddBCtr/1 -> Delay2/1
  [IM2] -> Delay12/1
  Delay13/1 -> AddBCtr/2, Delay4/1
  Delay8/1 -> Delay6/1
  Delay1/1 -> Delay7/1
  Delay12/1 -> Delay3/1
  Delay4/1 -> Delay23/1
  Delay5/1 -> Delay24/1
  Delay6/1 -> Product/1
  Delay2/1 -> Delay21/1
  Delay3/1 -> Delay22/1
  Delay23/1 -> Product2/1
  Delay24/1 -> Product2/2
  Delay21/1 -> Product1/1
  Delay22/1 -> Product1/2
  Delay25/1 -> Delay16/1
  Delay27/1 -> Delay18/1
  Delay16/1 -> AddAUp/1
  Delay26/1 -> Delay17/1
  Delay17/1 -> AddAUp/2, AddADn/1
  Delay20/1 -> Real-Imag to Complex/2
  Real-Imag to Complex/1 -> Out1/1

== system gm_soc_dvbs2_fpga/DVBS2/DVBS2 TxRx/DVB-S2 HDL Receiver/Synchronizer and PL Header Decoder/Time Frequency and Coarse Phase Synchronizer/Fine Frequency Synchronizer/Modified L and R Algorithm/L and R Algorithm 18 point/Compute R(m) for 1 to 6/Compute R(m)_4/Complex Multiplier ==
  In1 : Inport  OutDataTypeStr=fixdt(1, 16, 11)  PortDimensions=1  SampleTime=2.5e-07
      settings: SignalType=complex
  In2 : Inport  Port=2  OutDataTypeStr=fixdt(1, 16, 11)  PortDimensions=1  SampleTime=2.5e-07
      settings: SignalType=complex
  AddADn : Sum  Inputs=++|  OutDataTypeStr=fixdt(1, 33, 22)
  AddAUp : Sum  Inputs=|+-  OutDataTypeStr=fixdt(1, 33, 22)
  AddBCtr : Sum  Inputs=+|+  OutDataTypeStr=fixdt(1, 17, 11)
  AddBDn : Sum  Inputs=|+-  OutDataTypeStr=fixdt(1, 17, 11)
  AddBUp : Sum  Inputs=++|  OutDataTypeStr=fixdt(1, 17, 11)
  Complex to Real-Imag : ComplexToRealImag
  Complex to Real-Imag1 : ComplexToRealImag
  Delay{1..5,8..20} (18 alike) : Delay  DelayLength=1
  Delay{6..7,21..27} (9 alike) : Delay
  Product : Product  OutDataTypeStr=fixdt(1, 33, 22)
  Product1 : Product  OutDataTypeStr=fixdt(1, 33, 22)
  Product2 : Product  OutDataTypeStr=fixdt(1, 33, 22)
  Real-Imag to Complex : RealImagToComplex
  Out1 : Outport  SampleTime=2.5e-07  VectorParamsAs1DForOutWhenUnconnected=off
  wires:
  Delay9/1 -> AddBUp/1
  Delay7/1 -> Product/2
  [IM2] -> Delay15/1
  Delay26/1 -> Delay17/1
  [RE2] -> Delay14/1
  Delay5/1 -> Delay24/1
  [IM2] -> Delay10/1
  Product/1 -> Delay25/1
  Delay24/1 -> Product2/2
  [RE2] -> Delay9/1
  Delay11/1 -> AddBCtr/1, Delay1/1
  In1/1 -> Complex to Real-Imag/1
  Delay18/1 -> AddADn/2
  Delay10/1 -> AddBUp/2
  Delay12/1 -> Delay3/1
  In2/1 -> Complex to Real-Imag1/1
  Complex to Real-Imag/1 -> Delay11/1
  AddAUp/1 -> Delay19/1
  Complex to Real-Imag/2 -> Delay13/1
  Complex to Real-Imag1/1 -> [RE2]
  AddBCtr/1 -> Delay2/1
  Complex to Real-Imag1/2 -> [IM2]
  Delay14/1 -> AddBDn/1
  Delay15/1 -> AddBDn/2
  AddADn/1 -> Delay20/1
  AddBUp/1 -> Delay8/1
  Product1/1 -> Delay26/1
  [IM2] -> Delay12/1
  Delay13/1 -> AddBCtr/2, Delay4/1
  Real-Imag to Complex/1 -> Out1/1
  Product2/1 -> Delay27/1
  AddBDn/1 -> Delay5/1
  Delay8/1 -> Delay6/1
  Delay1/1 -> Delay7/1
  Delay4/1 -> Delay23/1
  Delay6/1 -> Product/1
  Delay2/1 -> Delay21/1
  Delay3/1 -> Delay22/1
  Delay23/1 -> Product2/1
  Delay21/1 -> Product1/1
  Delay22/1 -> Product1/2
  Delay25/1 -> Delay16/1
  Delay27/1 -> Delay18/1
  Delay16/1 -> AddAUp/1
  Delay17/1 -> AddAUp/2, AddADn/1
  Delay19/1 -> Real-Imag to Complex/1
  Delay20/1 -> Real-Imag to Complex/2

== system gm_soc_dvbs2_fpga/DVBS2/DVBS2 TxRx/DVB-S2 HDL Receiver/Synchronizer and PL Header Decoder/Time Frequency and Coarse Phase Synchronizer/Fine Frequency Synchronizer/Modified L and R Algorithm/L and R Algorithm 18 point/Compute R(m) for 1 to 6/Compute R(m)_5/Complex Multiplier ==
  In1 : Inport  OutDataTypeStr=fixdt(1, 16, 11)  PortDimensions=1  SampleTime=2.5e-07
      settings: SignalType=complex
  In2 : Inport  Port=2  OutDataTypeStr=fixdt(1, 16, 11)  PortDimensions=1  SampleTime=2.5e-07
      settings: SignalType=complex
  AddADn : Sum  Inputs=++|  OutDataTypeStr=fixdt(1, 33, 22)
  AddAUp : Sum  Inputs=|+-  OutDataTypeStr=fixdt(1, 33, 22)
  AddBCtr : Sum  Inputs=+|+  OutDataTypeStr=fixdt(1, 17, 11)
  AddBDn : Sum  Inputs=|+-  OutDataTypeStr=fixdt(1, 17, 11)
  AddBUp : Sum  Inputs=++|  OutDataTypeStr=fixdt(1, 17, 11)
  Complex to Real-Imag : ComplexToRealImag
  Complex to Real-Imag1 : ComplexToRealImag
  Delay{1..5,8..20} (18 alike) : Delay  DelayLength=1
  Delay{6..7,21..27} (9 alike) : Delay
  Product : Product  OutDataTypeStr=fixdt(1, 33, 22)
  Product1 : Product  OutDataTypeStr=fixdt(1, 33, 22)
  Product2 : Product  OutDataTypeStr=fixdt(1, 33, 22)
  Real-Imag to Complex : RealImagToComplex
  Out1 : Outport  SampleTime=2.5e-07  VectorParamsAs1DForOutWhenUnconnected=off
  wires:
  Delay9/1 -> AddBUp/1
  Real-Imag to Complex/1 -> Out1/1
  Product2/1 -> Delay27/1
  AddBDn/1 -> Delay5/1
  [IM2] -> Delay15/1
  [RE2] -> Delay14/1
  [IM2] -> Delay10/1
  AddAUp/1 -> Delay19/1
  Product/1 -> Delay25/1
  Complex to Real-Imag/2 -> Delay13/1
  [RE2] -> Delay9/1
  In1/1 -> Complex to Real-Imag/1
  In2/1 -> Complex to Real-Imag1/1
  Delay18/1 -> AddADn/2
  Delay10/1 -> AddBUp/2
  Complex to Real-Imag/1 -> Delay11/1
  Complex to Real-Imag1/1 -> [RE2]
  Product1/1 -> Delay26/1
  AddBCtr/1 -> Delay2/1
  [IM2] -> Delay12/1
  Complex to Real-Imag1/2 -> [IM2]
  Delay14/1 -> AddBDn/1
  Delay15/1 -> AddBDn/2
  AddADn/1 -> Delay20/1
  AddBUp/1 -> Delay8/1
  Delay19/1 -> Real-Imag to Complex/1
  Delay11/1 -> AddBCtr/1, Delay1/1
  Delay13/1 -> AddBCtr/2, Delay4/1
  Delay8/1 -> Delay6/1
  Delay1/1 -> Delay7/1
  Delay12/1 -> Delay3/1
  Delay4/1 -> Delay23/1
  Delay5/1 -> Delay24/1
  Delay6/1 -> Product/1
  Delay7/1 -> Product/2
  Delay2/1 -> Delay21/1
  Delay3/1 -> Delay22/1
  Delay23/1 -> Product2/1
  Delay24/1 -> Product2/2
  Delay21/1 -> Product1/1
  Delay22/1 -> Product1/2
  Delay25/1 -> Delay16/1
  Delay27/1 -> Delay18/1
  Delay16/1 -> AddAUp/1
  Delay26/1 -> Delay17/1
  Delay17/1 -> AddAUp/2, AddADn/1
  Delay20/1 -> Real-Imag to Complex/2

== system gm_soc_dvbs2_fpga/DVBS2/DVBS2 TxRx/DVB-S2 HDL Receiver/Synchronizer and PL Header Decoder/Time Frequency and Coarse Phase Synchronizer/Fine Frequency Synchronizer/Modified L and R Algorithm/L and R Algorithm 18 point/Compute R(m) for 1 to 6/Compute R(m)_6/Complex Multiplier ==
  In1 : Inport  OutDataTypeStr=fixdt(1, 16, 11)  PortDimensions=1  SampleTime=2.5e-07
      settings: SignalType=complex
  In2 : Inport  Port=2  OutDataTypeStr=fixdt(1, 16, 11)  PortDimensions=1  SampleTime=2.5e-07
      settings: SignalType=complex
  AddADn : Sum  Inputs=++|  OutDataTypeStr=fixdt(1, 33, 22)
  AddAUp : Sum  Inputs=|+-  OutDataTypeStr=fixdt(1, 33, 22)
  AddBCtr : Sum  Inputs=+|+  OutDataTypeStr=fixdt(1, 17, 11)
  AddBDn : Sum  Inputs=|+-  OutDataTypeStr=fixdt(1, 17, 11)
  AddBUp : Sum  Inputs=++|  OutDataTypeStr=fixdt(1, 17, 11)
  Complex to Real-Imag : ComplexToRealImag
  Complex to Real-Imag1 : ComplexToRealImag
  Delay{1..5,8..20} (18 alike) : Delay  DelayLength=1
  Delay{6..7,21..27} (9 alike) : Delay
  Product : Product  OutDataTypeStr=fixdt(1, 33, 22)
  Product1 : Product  OutDataTypeStr=fixdt(1, 33, 22)
  Product2 : Product  OutDataTypeStr=fixdt(1, 33, 22)
  Real-Imag to Complex : RealImagToComplex
  Out1 : Outport  SampleTime=2.5e-07  VectorParamsAs1DForOutWhenUnconnected=off
  wires:
  Delay9/1 -> AddBUp/1
  Product2/1 -> Delay27/1
  Delay7/1 -> Product/2
  [IM2] -> Delay15/1
  Delay26/1 -> Delay17/1
  [RE2] -> Delay14/1
  Delay5/1 -> Delay24/1
  [IM2] -> Delay10/1
  Product/1 -> Delay25/1
  Delay24/1 -> Product2/2
  [RE2] -> Delay9/1
  Delay19/1 -> Real-Imag to Complex/1
  Delay11/1 -> AddBCtr/1, Delay1/1
  In1/1 -> Complex to Real-Imag/1
  Delay18/1 -> AddADn/2
  Delay10/1 -> AddBUp/2
  Delay12/1 -> Delay3/1
  In2/1 -> Complex to Real-Imag1/1
  Complex to Real-Imag/1 -> Delay11/1
  AddAUp/1 -> Delay19/1
  Complex to Real-Imag/2 -> Delay13/1
  Complex to Real-Imag1/1 -> [RE2]
  AddBCtr/1 -> Delay2/1
  Complex to Real-Imag1/2 -> [IM2]
  Delay14/1 -> AddBDn/1
  Delay15/1 -> AddBDn/2
  AddBUp/1 -> Delay8/1
  Product1/1 -> Delay26/1
  [IM2] -> Delay12/1
  Delay13/1 -> AddBCtr/2, Delay4/1
  Real-Imag to Complex/1 -> Out1/1
  AddBDn/1 -> Delay5/1
  Delay8/1 -> Delay6/1
  Delay1/1 -> Delay7/1
  Delay4/1 -> Delay23/1
  Delay6/1 -> Product/1
  Delay2/1 -> Delay21/1
  AddADn/1 -> Delay20/1
  Delay3/1 -> Delay22/1
  Delay23/1 -> Product2/1
  Delay21/1 -> Product1/1
  Delay22/1 -> Product1/2
  Delay25/1 -> Delay16/1
  Delay27/1 -> Delay18/1
  Delay16/1 -> AddAUp/1
  Delay17/1 -> AddADn/1, AddAUp/2
  Delay20/1 -> Real-Imag to Complex/2

== system gm_soc_dvbs2_fpga/DVBS2/DVBS2 TxRx/DVB-S2 HDL Receiver/Synchronizer and PL Header Decoder/Time Frequency and Coarse Phase Synchronizer/Fine Frequency Synchronizer/Modified L and R Algorithm/L and R Algorithm 18 point/Compute R(m) for 13 to 18/Compute R(m)_1/Complex Multiplier ==
  In1 : Inport  OutDataTypeStr=fixdt(1, 16, 11)  PortDimensions=1  SampleTime=2.5e-07
      settings: SignalType=complex
  In2 : Inport  Port=2  OutDataTypeStr=fixdt(1, 16, 11)  PortDimensions=1  SampleTime=2.5e-07
      settings: SignalType=complex
  AddADn : Sum  Inputs=++|  OutDataTypeStr=fixdt(1, 33, 22)
  AddAUp : Sum  Inputs=|+-  OutDataTypeStr=fixdt(1, 33, 22)
  AddBCtr : Sum  Inputs=+|+  OutDataTypeStr=fixdt(1, 17, 11)
  AddBDn : Sum  Inputs=|+-  OutDataTypeStr=fixdt(1, 17, 11)
  AddBUp : Sum  Inputs=++|  OutDataTypeStr=fixdt(1, 17, 11)
  Complex to Real-Imag : ComplexToRealImag
  Complex to Real-Imag1 : ComplexToRealImag
  Delay{1..5,8..20} (18 alike) : Delay  DelayLength=1
  Delay{6..7,21..27} (9 alike) : Delay
  Product : Product  OutDataTypeStr=fixdt(1, 33, 22)
  Product1 : Product  OutDataTypeStr=fixdt(1, 33, 22)
  Product2 : Product  OutDataTypeStr=fixdt(1, 33, 22)
  Real-Imag to Complex : RealImagToComplex
  Out1 : Outport  SampleTime=2.5e-07  VectorParamsAs1DForOutWhenUnconnected=off
  wires:
  Real-Imag to Complex/1 -> Out1/1
  Product2/1 -> Delay27/1
  AddBDn/1 -> Delay5/1
  [IM2] -> Delay15/1
  [RE2] -> Delay14/1
  [IM2] -> Delay10/1
  AddAUp/1 -> Delay19/1
  Product/1 -> Delay25/1
  Complex to Real-Imag/2 -> Delay13/1
  [RE2] -> Delay9/1
  In1/1 -> Complex to Real-Imag/1
  Complex to Real-Imag/1 -> Delay11/1
  In2/1 -> Complex to Real-Imag1/1
  Delay19/1 -> Real-Imag to Complex/1
  Delay9/1 -> AddBUp/1
  Delay10/1 -> AddBUp/2
  Complex to Real-Imag1/1 -> [RE2]
  Product1/1 -> Delay26/1
  AddBCtr/1 -> Delay2/1
  [IM2] -> Delay12/1
  Complex to Real-Imag1/2 -> [IM2]
  Delay14/1 -> AddBDn/1
  Delay5/1 -> Delay24/1
  Delay15/1 -> AddBDn/2
  AddADn/1 -> Delay20/1
  AddBUp/1 -> Delay8/1
  Delay11/1 -> AddBCtr/1, Delay1/1
  Delay13/1 -> AddBCtr/2, Delay4/1
  Delay18/1 -> AddADn/2
  Delay8/1 -> Delay6/1
  Delay1/1 -> Delay7/1
  Delay12/1 -> Delay3/1
  Delay4/1 -> Delay23/1
  Delay16/1 -> AddAUp/1
  Delay6/1 -> Product/1
  Delay17/1 -> AddADn/1, AddAUp/2
  Delay7/1 -> Product/2
  Delay2/1 -> Delay21/1
  Delay3/1 -> Delay22/1
  Delay23/1 -> Product2/1
  Delay24/1 -> Product2/2
  Delay21/1 -> Product1/1
  Delay22/1 -> Product1/2
  Delay25/1 -> Delay16/1
  Delay27/1 -> Delay18/1
  Delay26/1 -> Delay17/1
  Delay20/1 -> Real-Imag to Complex/2

== system gm_soc_dvbs2_fpga/DVBS2/DVBS2 TxRx/DVB-S2 HDL Receiver/Synchronizer and PL Header Decoder/Time Frequency and Coarse Phase Synchronizer/Fine Frequency Synchronizer/Modified L and R Algorithm/L and R Algorithm 18 point/Compute R(m) for 13 to 18/Compute R(m)_2/Complex Multiplier ==
  In1 : Inport  OutDataTypeStr=fixdt(1, 16, 11)  PortDimensions=1  SampleTime=2.5e-07
      settings: SignalType=complex
  In2 : Inport  Port=2  OutDataTypeStr=fixdt(1, 16, 11)  PortDimensions=1  SampleTime=2.5e-07
      settings: SignalType=complex
  AddADn : Sum  Inputs=++|  OutDataTypeStr=fixdt(1, 33, 22)
  AddAUp : Sum  Inputs=|+-  OutDataTypeStr=fixdt(1, 33, 22)
  AddBCtr : Sum  Inputs=+|+  OutDataTypeStr=fixdt(1, 17, 11)
  AddBDn : Sum  Inputs=|+-  OutDataTypeStr=fixdt(1, 17, 11)
  AddBUp : Sum  Inputs=++|  OutDataTypeStr=fixdt(1, 17, 11)
  Complex to Real-Imag : ComplexToRealImag
  Complex to Real-Imag1 : ComplexToRealImag
  Delay{1..5,8..20} (18 alike) : Delay  DelayLength=1
  Delay{6..7,21..27} (9 alike) : Delay
  Product : Product  OutDataTypeStr=fixdt(1, 33, 22)
  Product1 : Product  OutDataTypeStr=fixdt(1, 33, 22)
  Product2 : Product  OutDataTypeStr=fixdt(1, 33, 22)
  Real-Imag to Complex : RealImagToComplex
  Out1 : Outport  SampleTime=2.5e-07  VectorParamsAs1DForOutWhenUnconnected=off
  wires:
  Delay9/1 -> AddBUp/1
  Product2/1 -> Delay27/1
  Delay7/1 -> Product/2
  [IM2] -> Delay15/1
  Delay26/1 -> Delay17/1
  [RE2] -> Delay14/1
  Delay5/1 -> Delay24/1
  [IM2] -> Delay10/1
  AddAUp/1 -> Delay19/1
  Product/1 -> Delay25/1
  [RE2] -> Delay9/1
  Delay19/1 -> Real-Imag to Complex/1
  Delay11/1 -> Delay1/1, AddBCtr/1
  In1/1 -> Complex to Real-Imag/1
  Delay18/1 -> AddADn/2
  Delay10/1 -> AddBUp/2
  Delay12/1 -> Delay3/1
  In2/1 -> Complex to Real-Imag1/1
  Complex to Real-Imag/1 -> Delay11/1
  Complex to Real-Imag/2 -> Delay13/1
  Complex to Real-Imag1/1 -> [RE2]
  AddBCtr/1 -> Delay2/1
  Complex to Real-Imag1/2 -> [IM2]
  Delay14/1 -> AddBDn/1
  Delay15/1 -> AddBDn/2
  AddBUp/1 -> Delay8/1
  Product1/1 -> Delay26/1
  [IM2] -> Delay12/1
  Delay13/1 -> AddBCtr/2, Delay4/1
  Real-Imag to Complex/1 -> Out1/1
  AddBDn/1 -> Delay5/1
  Delay8/1 -> Delay6/1
  Delay1/1 -> Delay7/1
  Delay4/1 -> Delay23/1
  Delay6/1 -> Product/1
  Delay2/1 -> Delay21/1
  AddADn/1 -> Delay20/1
  Delay3/1 -> Delay22/1
  Delay23/1 -> Product2/1
  Delay24/1 -> Product2/2
  Delay21/1 -> Product1/1
  Delay22/1 -> Product1/2
  Delay25/1 -> Delay16/1
  Delay27/1 -> Delay18/1
  Delay16/1 -> AddAUp/1
  Delay17/1 -> AddAUp/2, AddADn/1
  Delay20/1 -> Real-Imag to Complex/2
